simulink model "QPSK_iid_Rayleigh"  (R2019b)
settings: Solver=VariableStepAuto  StartTime=0.0  StopTime=0.01  RelTol=1e-3
libraries: commutil2 x2, commdigbbndpm3 x2, commchan3 x1, commrandsrc3 x1, commsink2 x1
settings Model: Creator=Nikhil  LastModifiedBy=Nikhil

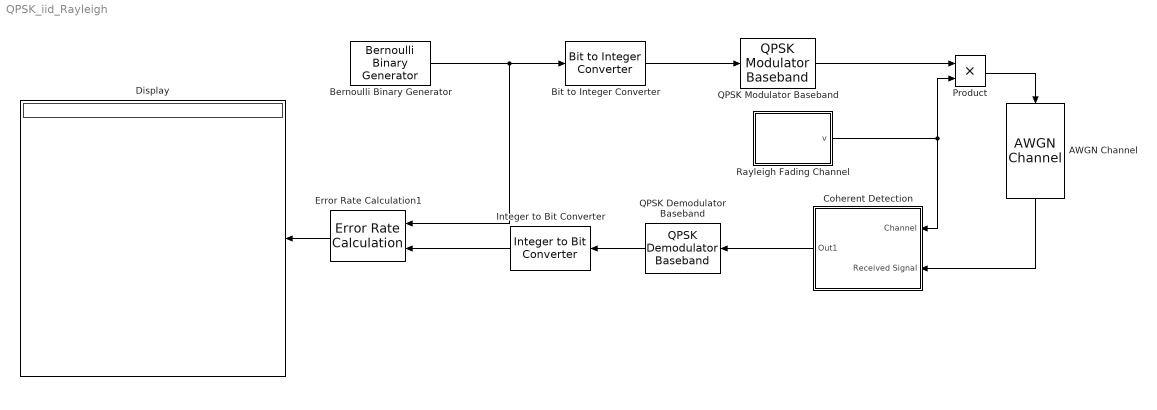
== system QPSK_iid_Rayleigh ==
  AWGN Channel : commchan3/AWGN Channel  InputProcessing=Columns as channels (frame based)  seed=117  noiseMode="Signal to noise ratio  (SNR)"  EbNodB=10  EsNodB=10  SNRdB=12  bitsPerSym=2  Ps=1  Tsym=5e-7  variance=1
      settings: SourceProductName=Communications Toolbox
  Bernoulli Binary Generator : commrandsrc3/Bernoulli Binary Generator  ProbabilityOfZero=0.5  SeedSource=Parameter  Seed=322  SampleTime=1e-6  SamplesPerFrame=2  OutputDataType=uint8  SimulateUsing=Interpreted execution
      settings: SourceProductName=Communications Toolbox
  Bit to Integer Converter : commutil2/Bit to Integer Converter  nbits=2  bitOrder=MSB first  signedOutputValues=Unsigned  outDtype=Inherit via internal rule  outDtypeSigned=Inherit via internal rule
      settings: SourceProductName=Communications Toolbox
  Coherent Detection : Subsystem
  Display : Display
  Error Rate Calculation1 : commsink2/Error Rate Calculation  N=0  st_delay=0  cp_mode=Entire frame  subframe=[]  PMode=Port  WsName=ErrorVec  RsMode2=off  stop=off  numErr=100  maxBits=1e6
      settings: SourceProductName=Communications Toolbox
  Integer to Bit Converter : commutil2/Integer to Bit Converter  nbits=2  signedInputValues=Unsigned  bitOrder=MSB first  outDtype=Inherit via internal rule
      settings: SourceProductName=Communications Toolbox
  Product : Product
  QPSK Demodulator Baseband : commdigbbndpm3/QPSK Demodulator Baseband  OutType=Integer  DecType=Hard decision  VarSource=Dialog  Variance=1  Dec=Gray  Ph=pi/4  outDtype1=Inherit via internal rule  outDtype2=Inherit via internal rule  derotateFactorWordLen=16  derotateFactorDataTypeStr=Inherit: Same word length as input  derotateFactorLastDataTypeStr=Inherit: Same word length as input
      settings: SourceProductName=Communications Toolbox
  QPSK Modulator Baseband : commdigbbndpm3/QPSK Modulator Baseband  InType=Integer  Enc=Gray  Ph=pi/4  outDtype=Inherit via back propagation  outWordLen=16  outUDDataType=sfix(16)  outFracLenMode=Best precision  outFracLen=15  outDataTypeStr=Inherit: Inherit via back propagation  outLastDataTypeStr=Inherit: Inherit via back propagation
      settings: SourceProductName=Communications Toolbox
  Rayleigh Fading Channel : Subsystem
  wires:
  Bit to Integer Converter/1 -> QPSK Modulator Baseband/1
  Product/1 -> AWGN Channel/1
  QPSK Modulator Baseband/1 -> Product/1
  Integer to Bit Converter/1 -> Error Rate Calculation1/2
  QPSK Demodulator Baseband/1 -> Integer to Bit Converter/1
  Rayleigh Fading Channel/1(v) -> Coherent Detection/1(Channel), Product/2
  AWGN Channel/1 -> Coherent Detection/2(Received Signal)
  Coherent Detection/1(Out1) -> QPSK Demodulator Baseband/1
  Bernoulli Binary Generator/1 -> Error Rate Calculation1/1, Bit to Integer Converter/1
  Error Rate Calculation1/1 -> Display/1

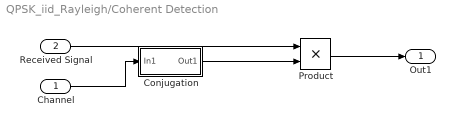
== system QPSK_iid_Rayleigh/Coherent Detection ==
  Channel : Inport
  Received Signal : Inport  Port=2
  Conjugation : Subsystem
  Product : Product
  Out1 : Outport
  wires:
  Channel/1 -> Conjugation/1(In1)
  Product/1 -> Out1/1
  Received Signal/1 -> Product/1
  Conjugation/1(Out1) -> Product/2

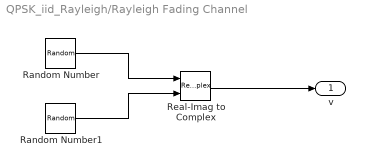
== system QPSK_iid_Rayleigh/Rayleigh Fading Channel ==
  Random Number : RandomNumber  Variance=1/2  Seed=420  SampleTime=1e-6
  Random Number1 : RandomNumber  Variance=1/2  Seed=69  SampleTime=1e-6
  Real-Imag to Complex : RealImagToComplex
  v : Outport
  wires:
  Real-Imag to Complex/1 -> v/1
  Random Number/1 -> Real-Imag to Complex/1
  Random Number1/1 -> Real-Imag to Complex/2

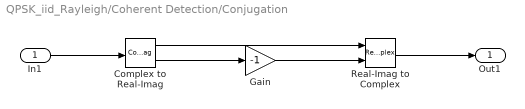
== system QPSK_iid_Rayleigh/Coherent Detection/Conjugation ==
  In1 : Inport
  Complex to Real-Imag : ComplexToRealImag
  Gain : Gain  Gain=-1
  Real-Imag to Complex : RealImagToComplex
  Out1 : Outport
  wires:
  In1/1 -> Complex to Real-Imag/1
  Complex to Real-Imag/1 -> Real-Imag to Complex/1
  Complex to Real-Imag/2 -> Gain/1
  Gain/1 -> Real-Imag to Complex/2
  Real-Imag to Complex/1 -> Out1/1
